simulink library "ME598_ProjectLibrary"  (R2025a)
settings: Solver=ode23t  StartTime=0.0  StopTime=10.0  RelTol=1e-3
InitFcn:
  | RPInit
undefined symbols (not defined in the file or in its folder): Base, FloorSurface, PlowSurface, Ref, RobotSurface, Side1, Side2, X, Y, Z
libraries: sm_lib x27, nesl_utility x11, RoboticsPlayground x8, RP_Simulator_Components x7, robotmobilelib x1
(part 2 of 2)

== matlab function ME598_ProjectLibrary/Object Detector/See Blue/MATLAB Function ==
  data: objectsDetected input size=[5 3]; angle output; range output; color parameter
function [angle,range] = pickColor(objectsDetected, color)
%#codegen

if ~isempty(objectsDetected)
    colorDetections=objectsDetected(:,3)==color;
    if any(colorDetections)
        colorObjects=objectsDetected(colorDetections,1:2);
        angle=colorObjects(1,2);
        range=colorObjects(1,1);
    else
        angle=NaN;
        range=NaN;
    end
else
    angle=NaN;
    range=NaN;
end
